simulink model "digitaltwin1c"  (R2020a)
settings: Solver=VariableStepAuto  StartTime=0.0  StopTime=stoptimetotal  RelTol=1e-3
values from neighbouring files (symbols this model uses):
  IC = load('params/IC_HoverAt10ftOcto.mat').IC    [prognostics.m]    (also in workspace_1.mat = )
  Motortwin1 = load('params/Motors/Motor1.mat').Motor    [prognostics.m]    (also in workspace_1.mat = )
  Motortwin2 = load('params/Motors/Motor2.mat').Motor    [prognostics.m]    (also in workspace_1.mat = )
  Motortwin3 = load('params/Motors/Motor3.mat').Motor    [prognostics.m]    (also in workspace_1.mat = )
  Motortwin4 = load('params/Motors/Motor4.mat').Motor    [prognostics.m]    (also in workspace_1.mat = )
  Motortwin5 = load('params/Motors/Motor5.mat').Motor    [prognostics.m]    (also in workspace_1.mat = )
  Motortwin6 = load('params/Motors/Motor6.mat').Motor    [prognostics.m]    (also in workspace_1.mat = )
  Motortwin7 = load('params/Motors/Motor7.mat').Motor    [prognostics.m]    (also in workspace_1.mat = )
  Motortwin8 = load('params/Motors/Motor8.mat').Motor    [prognostics.m]    (also in workspace_1.mat = )
  octomodel = load('params/octoModel.mat').octomodel    [prognostics.m]    (also in workspace_1.mat = )
  sampletimetraj = 1    [prognostics.m]    (also in workspace_1.mat)
undefined symbols (not defined in the file or in its folder): DiscIntNeverNeededParam, mu_wind
libraries: simulink x1, dspstat3 x1
(part 2 of 2)

== matlab function digitaltwin1c/Control allocation ==
  data: Fx input; wref1 output; Fy input; Fz input; Troll input; Tpitch input; Tyaw input; wref2 output; wref3 output; wref4 output; wref5 output; wref6 output; wref7 output; wref8 output
function [wref1,wref2,wref3,wref4,wref5,wref6,wref7,wref8] = fcn(Fx,Fy,Fz,Troll,Tpitch,Tyaw)
%% parameters 
%Maximum speed that the motors can reach in rad/s, if I check voltage, I
%dont have to check speed
% Max_speed=710.31;
Max_speed=1000;

% arm length - distances from the octorotor center of mass ...
%        to the center of mass of all its rotors are equal and denoted by l.
l=0.35;
% thrust motor constant [Ns^2/rad^2]
b=8.54858e-06; % cq
% rotor drag constant [Nms^2/rad^2]
d=1.3678e-07; % ct
% control allocation matrix
A_f=[2*b 2*b 2*b 2*b; ...
    b*l 0 -b*l 0; ...
    -b*l -sqrt(2)*b*l b*l sqrt(2)*b*l; ...
    -2*d 2*d -2*d 2*d];
%desired input
u_des=[Fz;Troll;Tpitch;Tyaw];

%control allocation
Omega_sf=inv(A_f)*u_des;

%selection operator
E=[1 0 1 0 0 0 0 0;...
    0 1 0 1 0 0 0 0; ...
    0 0 0 0 1 0 1 0;...
    0 0 0 0 0 1 0 1]';

Omega_s=E*Omega_sf;

% velocity checking
wref=zeros(8);
for i=1:length(Omega_s)
    if Omega_s(i)<0
        wref(i)=0;
    elseif Omega_s(i)>Max_speed^2
        wref(i)=Max_speed;
    else
        wref(i)=sqrt(Omega_s(i));
    end
end

%velocity assignment in V
multiply=0.012240; %for 6783 rpm considering torque load 
for i=1:length(wref)
    % voltage saturation check
    if(wref(i)*multiply > 11.1)
        wref(i)=11.1;
    else
        wref(i)=wref(i)*multiply;
    end
end

wref1=wref(1);
wref2=wref(2);
wref3=wref(3);
wref4=wref(4);
wref5=wref(5);
wref6=wref(6);
wref7=wref(7);
wref8=wref(8);







% %% parameters required
% % load('params/octoModel.mat');
% gamma=3;%octomodel.tiltmotorangle;
% alpha=45;%octomodel.separationmotorangle;
% dl=0.45;%octomodel.dl;
% constant=(1/sqrt(2));
% ds=0.35;%octomodel.ds;
% ct=3.4262e-05;%octomodel.ct*(60/(2*pi))^2 -> in octomodel is for rpm, here I need it in rad/s;
% cq=9.3846e-07;%octomodel.cq*(60/(2*pi))^2 -> in octomodel is for rpm, here I need it in rad/s;
% 
% %% rotation matrices because of 3 degrees tilted angle
% 
% E_m_b = [0 -sin(alpha)*sin(gamma) sin(gamma) -cos(alpha)*sin(gamma) 0 sin(alpha)*sin(gamma) -sin(gamma) cos(alpha)*sin(gamma);
%          -sin(gamma)  cos(alpha)*sin(gamma) 0 -sin(alpha)*sin(gamma) sin(gamma) -cos(alpha)*sin(gamma) 0 sin(alpha)*sin(gamma);
%          -cos(gamma) -cos(gamma) -cos(gamma) -cos(gamma) -cos(gamma) -cos(gamma) -cos(gamma) -cos(gamma)];
% 
% R_m=[dl 0 0; ...
%     constant*ds constant*ds 0; ...
%     0 dl 0; ...
%     -constant*ds constant*ds 0; ...
%     -dl 0 0; ...
%     -constant*ds -constant*ds 0; ...
%     0 -dl 0; ...
%     constant*ds -constant*ds 0]';
% 
% %% first form delta_b matrix
% %a vectors
% a=zeros(3,8);
% for i=1:8
%     e_i_b=E_m_b(:,i);
%     a(:,i)=(ct).*e_i_b;
% end
% 
% %b vectors
% b=zeros(3,8);
% for i=1:8
%     e_i_b=E_m_b(:,i);
%     r_m=R_m(:,i);
%     b(:,i)=cross( r_m,(ct).*e_i_b ) + ((-1)^(i+1)*(cq)).*e_i_b;    
% end
% 
% %form matrix
% delta_b=[a;b];
% 
% %find pseudo-inverse
% delta_binv = pinv(delta_b);
% 
% %% calculate required w_ref
% Forces=[Fx,Fy,Fz];
% Torques=[Troll,Tpitch,Tyaw];
% if Troll>0
%     see=1;
% end
% input=[Forces,Torques]';
% wref=delta_binv*input;
% %check if complex
% if(isreal(wref(2)))
%     see=1;
% end
% 
% if length(find(wref<0))>0
%     pos=find(wref<0);
%     wref(pos)=0;
% end
% wref=sqrt(wref);
% 
% % %angular velocity in rad/s
% % wref1=wref(1);
% % wref2=wref(2);
% % wref3=wref(3);
% % wref4=wref(4);
% % wref5=wref(5);
% % wref6=wref(6);
% % wref7=wref(7);
% % wref8=wref(8);
% 
% %angular velocity in rpm
% % wref1=wref(1)*(60/(2*pi));
% % wref2=wref(2)*(60/(2*pi));
% % wref3=wref(3)*(60/(2*pi));
% % wref4=wref(4)*(60/(2*pi));
% % wref5=wref(5)*(60/(2*pi));
% % wref6=wref(6)*(60/(2*pi));
% % wref7=wref(7)*(60/(2*pi));
% % wref8=wref(8)*(60/(2*pi));
% 
% %% now convert to voltage in the range 0-22V
% % divide=36.17; %true is 36.37
% % multiply=0.0238; %for 8800 rpm nominal 
% multiply=0.02762; %for 6783 rpm considering torque load 
% wref1=wref(1)*multiply;
% wref2=wref(2)*multiply;
% wref3=wref(3)*multiply;
% wref4=wref(4)*multiply;
% wref5=wref(5)*multiply;
% wref6=wref(6)*multiply;
% wref7=wref(7)*multiply;
% wref8=wref(8)*multiply;
% 
% see=1;

end
